simulink model "VCU_CS75_12_16_Test"  (R2014a)
settings: Solver=FixedStepDiscrete  StartTime=0.0  StopTime=25  FixedStep=0.0005  RelTol=1e-3
undefined symbols (not defined in the file): ecucoder_acal, I_SW01_L, LaterlAngleCommand, LDW, RemoteAcclPosition
libraries: simulink x913, ec5744lib x39
(part 25 of 30)

== system VCU_CS75_12_16_Test/长安CS75底盘程序，20ms一次/Input/CAN1_Rx/EMS_205/ReceiveMessages/Subsystem/EMS ==
  input : Inport
  Demux : Demux  Outputs=8
  EMS_CheckSum_205_Ad : Sum
  EMS_CheckSum_205_Convert : DataTypeConversion  OutDataTypeStr=uint32
  EMS_CheckSum_205_F : Gain
  EMS_CheckSum_205_L : simulink/Logic and Bit Operations/Bitwise Operator  logicop=AND  UseBitMask=on  BitMask=240  BitMaskRealWorld=Stored Integer
  EMS_CheckSum_205_O : Constant  Value=0  OutDataTypeStr=single
  EMS_CheckSum_205_S : ArithShift  BitShiftNumber=4
  EMS_CheckSum_205_Sub : Subsystem
  EMS_CheckSum_205_sat : Saturate  UpperLimit=15  LowerLimit=0
  EMS_CheckSum_205cv : DataTypeConversion
  EMS_ESPTorqReuestAvailability_Ad : Sum
  EMS_ESPTorqReuestAvailability_Convert : DataTypeConversion  OutDataTypeStr=uint32
  EMS_ESPTorqReuestAvailability_F : Gain
  EMS_ESPTorqReuestAvailability_L : simulink/Logic and Bit Operations/Bitwise Operator  logicop=AND  UseBitMask=on  BitMask=2  BitMaskRealWorld=Stored Integer
  EMS_ESPTorqReuestAvailability_O : Constant  Value=0  OutDataTypeStr=single
  EMS_ESPTorqReuestAvailability_S : ArithShift  BitShiftNumber=1
  EMS_ESPTorqReuestAvailability_Sub : Subsystem
  EMS_ESPTorqReuestAvailability_sat : Saturate  UpperLimit=1  LowerLimit=0  OutDataTypeStr=Inherit: Inherit via back propagation
  EMS_ESPTorqReuestAvailabilitycv : DataTypeConversion
  EMS_FrictionalTorq_Ad : Sum
  EMS_FrictionalTorq_Convert : DataTypeConversion  OutDataTypeStr=uint32
  EMS_FrictionalTorq_F : Gain  Gain=0.001526
  EMS_FrictionalTorq_L : simulink/Logic and Bit Operations/Bitwise Operator  logicop=AND  UseBitMask=on  BitMask=65535  BitMaskRealWorld=Stored Integer
  EMS_FrictionalTorq_O : Constant  Value=0  OutDataTypeStr=single
  EMS_FrictionalTorq_S : ArithShift
  EMS_FrictionalTorq_Sub : Subsystem
  EMS_FrictionalTorq_sat : Saturate  UpperLimit=99.9988  LowerLimit=0
  EMS_FrictionalTorqcv : DataTypeConversion
  EMS_FrictionalTorqinput4_Ad : Sum
  EMS_FrictionalTorqinput4_C : Constant  Value=256
  EMS_FrictionalTorqinput4_P : Product
  EMS_IndicatedDriverReqTorq_Ad : Sum
  EMS_IndicatedDriverReqTorq_Convert : DataTypeConversion  OutDataTypeStr=uint32
  EMS_IndicatedDriverReqTorq_F : Gain  Gain=0.001526
  EMS_IndicatedDriverReqTorq_L : simulink/Logic and Bit Operations/Bitwise Operator  logicop=AND  UseBitMask=on  BitMask=65535  BitMaskRealWorld=Stored Integer
  EMS_IndicatedDriverReqTorq_O : Constant  Value=0  OutDataTypeStr=single
  EMS_IndicatedDriverReqTorq_S : ArithShift
  EMS_IndicatedDriverReqTorq_Sub : Subsystem
  EMS_IndicatedDriverReqTorq_sat : Saturate  UpperLimit=99.9988  LowerLimit=0
  EMS_IndicatedDriverReqTorqcv : DataTypeConversion
  EMS_IndicatedDriverReqTorqinput2_Ad : Sum
  EMS_IndicatedDriverReqTorqinput2_C : Constant  Value=256
  EMS_IndicatedDriverReqTorqinput2_P : Product
  EMS_IndicatedRealEngTorq_Ad : Sum
  EMS_IndicatedRealEngTorq_Convert : DataTypeConversion  OutDataTypeStr=uint32
  EMS_IndicatedRealEngTorq_F : Gain  Gain=0.001526
  EMS_IndicatedRealEngTorq_L : simulink/Logic and Bit Operations/Bitwise Operator  logicop=AND  UseBitMask=on  BitMask=65535  BitMaskRealWorld=Stored Integer
  EMS_IndicatedRealEngTorq_O : Constant  Value=0  OutDataTypeStr=single
  EMS_IndicatedRealEngTorq_S : ArithShift
  EMS_IndicatedRealEngTorq_Sub : Subsystem
  EMS_IndicatedRealEngTorq_sat : Saturate  UpperLimit=99.9988  LowerLimit=0
  EMS_IndicatedRealEngTorqcv : DataTypeConversion
  EMS_IndicatedRealEngTorqinput6_Ad : Sum
  EMS_IndicatedRealEngTorqinput6_C : Constant  Value=256
  EMS_IndicatedRealEngTorqinput6_P : Product
  EMS_RollingCounter_id205_Ad : Sum
  EMS_RollingCounter_id205_Convert : DataTypeConversion  OutDataTypeStr=uint32
  EMS_RollingCounter_id205_F : Gain
  EMS_RollingCounter_id205_L : simulink/Logic and Bit Operations/Bitwise Operator  logicop=AND  UseBitMask=on  BitMask=15  BitMaskRealWorld=Stored Integer
  EMS_RollingCounter_id205_O : Constant  Value=0  OutDataTypeStr=single
  EMS_RollingCounter_id205_S : ArithShift
  EMS_RollingCounter_id205_Sub : Subsystem
  EMS_RollingCounter_id205_sat : Saturate  UpperLimit=15  LowerLimit=0
  EMS_RollingCounter_id205cv : DataTypeConversion
  EMS_TorqFailure_Ad : Sum
  EMS_TorqFailure_Convert : DataTypeConversion  OutDataTypeStr=uint32
  EMS_TorqFailure_F : Gain
  EMS_TorqFailure_L : simulink/Logic and Bit Operations/Bitwise Operator  logicop=AND  UseBitMask=on  BitMask=128  BitMaskRealWorld=Stored Integer
  EMS_TorqFailure_O : Constant  Value=0  OutDataTypeStr=single
  EMS_TorqFailure_S : ArithShift  BitShiftNumber=7
  EMS_TorqFailure_Sub : Subsystem
  EMS_TorqFailure_sat : Saturate  UpperLimit=1  LowerLimit=0
  EMS_TorqFailurecv : DataTypeConversion
  EMS_ESPTorqReuestAvailability_Out : Outport
  EMS_TorqFailure_Out : Outport  Port=2
  EMS_IndicatedDriverReqTorq_Out : Outport  Port=3
  EMS_FrictionalTorq_Out : Outport  Port=4
  EMS_IndicatedRealEngTorq_Out : Outport  Port=5
  EMS_RollingCounter_id205_Out : Outport  Port=6
  EMS_CheckSum_205_Out : Outport  Port=7
  wires:
  EMS_ESPTorqReuestAvailability_F/1 -> EMS_ESPTorqReuestAvailability_Ad/1
  EMS_ESPTorqReuestAvailability_O/1 -> EMS_ESPTorqReuestAvailability_Ad/2
  EMS_ESPTorqReuestAvailability_sat/1 -> EMS_ESPTorqReuestAvailability_Out/1
  Demux/1 -> EMS_ESPTorqReuestAvailability_Sub/1(In1), EMS_TorqFailure_Sub/1(In1)
  EMS_ESPTorqReuestAvailability_Sub/1(Out1) -> EMS_ESPTorqReuestAvailability_Convert/1
  EMS_ESPTorqReuestAvailability_Convert/1 -> EMS_ESPTorqReuestAvailability_L/1
  EMS_ESPTorqReuestAvailability_L/1 -> EMS_ESPTorqReuestAvailability_S/1
  EMS_ESPTorqReuestAvailability_S/1 -> EMS_ESPTorqReuestAvailabilitycv/1
  EMS_ESPTorqReuestAvailabilitycv/1 -> EMS_ESPTorqReuestAvailability_F/1
  EMS_TorqFailure_F/1 -> EMS_TorqFailure_Ad/1
  EMS_TorqFailure_O/1 -> EMS_TorqFailure_Ad/2
  EMS_TorqFailure_Ad/1 -> EMS_TorqFailure_sat/1
  EMS_TorqFailure_sat/1 -> EMS_TorqFailure_Out/1
  EMS_TorqFailure_Sub/1(Out1) -> EMS_TorqFailure_Convert/1
  EMS_TorqFailure_Convert/1 -> EMS_TorqFailure_L/1
  EMS_TorqFailure_L/1 -> EMS_TorqFailure_S/1
  EMS_TorqFailure_S/1 -> EMS_TorqFailurecv/1
  EMS_TorqFailurecv/1 -> EMS_TorqFailure_F/1
  EMS_IndicatedDriverReqTorq_F/1 -> EMS_IndicatedDriverReqTorq_Ad/1
  EMS_IndicatedDriverReqTorq_O/1 -> EMS_IndicatedDriverReqTorq_Ad/2
  EMS_IndicatedDriverReqTorq_Ad/1 -> EMS_IndicatedDriverReqTorq_sat/1
  EMS_IndicatedDriverReqTorq_sat/1 -> EMS_IndicatedDriverReqTorq_Out/1
  Demux/2 -> EMS_IndicatedDriverReqTorqinput2_P/1
  EMS_IndicatedDriverReqTorqinput2_C/1 -> EMS_IndicatedDriverReqTorqinput2_P/2
  EMS_IndicatedDriverReqTorqinput2_P/1 -> EMS_IndicatedDriverReqTorqinput2_Ad/1
  Demux/3 -> EMS_IndicatedDriverReqTorqinput2_Ad/2
  EMS_IndicatedDriverReqTorqinput2_Ad/1 -> EMS_IndicatedDriverReqTorq_Sub/1(In1)
  EMS_IndicatedDriverReqTorq_Sub/1(Out1) -> EMS_IndicatedDriverReqTorq_Convert/1
  EMS_IndicatedDriverReqTorq_Convert/1 -> EMS_IndicatedDriverReqTorq_L/1
  EMS_IndicatedDriverReqTorq_L/1 -> EMS_IndicatedDriverReqTorq_S/1
  EMS_IndicatedDriverReqTorq_S/1 -> EMS_IndicatedDriverReqTorqcv/1
  EMS_IndicatedDriverReqTorqcv/1 -> EMS_IndicatedDriverReqTorq_F/1
  EMS_FrictionalTorq_F/1 -> EMS_FrictionalTorq_Ad/1
  EMS_FrictionalTorq_O/1 -> EMS_FrictionalTorq_Ad/2
  EMS_FrictionalTorq_Ad/1 -> EMS_FrictionalTorq_sat/1
  EMS_FrictionalTorq_sat/1 -> EMS_FrictionalTorq_Out/1
  Demux/4 -> EMS_FrictionalTorqinput4_P/1
  EMS_FrictionalTorqinput4_C/1 -> EMS_FrictionalTorqinput4_P/2
  EMS_FrictionalTorqinput4_P/1 -> EMS_FrictionalTorqinput4_Ad/1
  Demux/5 -> EMS_FrictionalTorqinput4_Ad/2
  EMS_FrictionalTorqinput4_Ad/1 -> EMS_FrictionalTorq_Sub/1(In1)
  EMS_FrictionalTorq_Sub/1(Out1) -> EMS_FrictionalTorq_Convert/1
  EMS_FrictionalTorq_Convert/1 -> EMS_FrictionalTorq_L/1
  EMS_FrictionalTorq_L/1 -> EMS_FrictionalTorq_S/1
  EMS_FrictionalTorq_S/1 -> EMS_FrictionalTorqcv/1
  EMS_FrictionalTorqcv/1 -> EMS_FrictionalTorq_F/1
  EMS_IndicatedRealEngTorq_F/1 -> EMS_IndicatedRealEngTorq_Ad/1
  EMS_IndicatedRealEngTorq_O/1 -> EMS_IndicatedRealEngTorq_Ad/2
  EMS_IndicatedRealEngTorq_Ad/1 -> EMS_IndicatedRealEngTorq_sat/1
  EMS_IndicatedRealEngTorq_sat/1 -> EMS_IndicatedRealEngTorq_Out/1
  Demux/6 -> EMS_IndicatedRealEngTorqinput6_P/1
  EMS_IndicatedRealEngTorqinput6_C/1 -> EMS_IndicatedRealEngTorqinput6_P/2
  EMS_IndicatedRealEngTorqinput6_P/1 -> EMS_IndicatedRealEngTorqinput6_Ad/1
  Demux/7 -> EMS_IndicatedRealEngTorqinput6_Ad/2
  EMS_IndicatedRealEngTorqinput6_Ad/1 -> EMS_IndicatedRealEngTorq_Sub/1(In1)
  EMS_IndicatedRealEngTorq_Sub/1(Out1) -> EMS_IndicatedRealEngTorq_Convert/1
  EMS_IndicatedRealEngTorq_Convert/1 -> EMS_IndicatedRealEngTorq_L/1
  EMS_IndicatedRealEngTorq_L/1 -> EMS_IndicatedRealEngTorq_S/1
  EMS_IndicatedRealEngTorq_S/1 -> EMS_IndicatedRealEngTorqcv/1
  EMS_IndicatedRealEngTorqcv/1 -> EMS_IndicatedRealEngTorq_F/1
  EMS_RollingCounter_id205_F/1 -> EMS_RollingCounter_id205_Ad/1
  EMS_RollingCounter_id205_O/1 -> EMS_RollingCounter_id205_Ad/2
  EMS_RollingCounter_id205_Ad/1 -> EMS_RollingCounter_id205_sat/1
  EMS_RollingCounter_id205_sat/1 -> EMS_RollingCounter_id205_Out/1
  Demux/8 -> EMS_RollingCounter_id205_Sub/1(In1), EMS_CheckSum_205_Sub/1(In1)
  EMS_RollingCounter_id205_Sub/1(Out1) -> EMS_RollingCounter_id205_Convert/1
  EMS_RollingCounter_id205_Convert/1 -> EMS_RollingCounter_id205_L/1
  EMS_RollingCounter_id205_L/1 -> EMS_RollingCounter_id205_S/1
  EMS_RollingCounter_id205_S/1 -> EMS_RollingCounter_id205cv/1
  EMS_RollingCounter_id205cv/1 -> EMS_RollingCounter_id205_F/1
  EMS_CheckSum_205_F/1 -> EMS_CheckSum_205_Ad/1
  EMS_CheckSum_205_O/1 -> EMS_CheckSum_205_Ad/2
  EMS_CheckSum_205_Ad/1 -> EMS_CheckSum_205_sat/1
  EMS_CheckSum_205_sat/1 -> EMS_CheckSum_205_Out/1
  EMS_CheckSum_205_Sub/1(Out1) -> EMS_CheckSum_205_Convert/1
  EMS_CheckSum_205_Convert/1 -> EMS_CheckSum_205_L/1
  EMS_CheckSum_205_L/1 -> EMS_CheckSum_205_S/1
  EMS_CheckSum_205_S/1 -> EMS_CheckSum_205cv/1
  EMS_CheckSum_205cv/1 -> EMS_CheckSum_205_F/1
  input/1 -> Demux/1
  EMS_ESPTorqReuestAvailability_Ad/1 -> EMS_ESPTorqReuestAvailability_sat/1

== system VCU_CS75_12_16_Test/长安CS75底盘程序，20ms一次/Input/CAN1_Rx/EMS_255/ReceiveMessages/Subsystem/EMS ==
  input : Inport
  Demux : Demux  Outputs=8
  EMS_AccPedal_Ad : Sum
  EMS_AccPedal_Convert : DataTypeConversion  OutDataTypeStr=uint32
  EMS_AccPedal_F : Gain  Gain=0.392
  EMS_AccPedal_L : simulink/Logic and Bit Operations/Bitwise Operator  logicop=AND  UseBitMask=on  BitMask=255  BitMaskRealWorld=Stored Integer
  EMS_AccPedal_O : Constant  Value=0  OutDataTypeStr=single
  EMS_AccPedal_S : ArithShift
  EMS_AccPedal_Sub : Subsystem
  EMS_AccPedal_sat : Saturate  UpperLimit=99.568  LowerLimit=0
  EMS_AccPedalcv : DataTypeConversion
  EMS_AccpedelError_Ad : Sum
  EMS_AccpedelError_Convert : DataTypeConversion  OutDataTypeStr=uint32
  EMS_AccpedelError_F : Gain
  EMS_AccpedelError_L : simulink/Logic and Bit Operations/Bitwise Operator  logicop=AND  UseBitMask=on  BitMask=4  BitMaskRealWorld=Stored Integer
  EMS_AccpedelError_O : Constant  Value=0  OutDataTypeStr=single
  EMS_AccpedelError_S : ArithShift  BitShiftNumber=2
  EMS_AccpedelError_Sub : Subsystem
  EMS_AccpedelError_sat : Saturate  UpperLimit=1  LowerLimit=0
  EMS_AccpedelErrorcv : DataTypeConversion
  EMS_BrakePedalStatus_Ad : Sum
  EMS_BrakePedalStatus_Convert : DataTypeConversion  OutDataTypeStr=uint32
  EMS_BrakePedalStatus_F : Gain
  EMS_BrakePedalStatus_L : simulink/Logic and Bit Operations/Bitwise Operator  logicop=AND  UseBitMask=on  BitMask=192  BitMaskRealWorld=Stored Integer
  EMS_BrakePedalStatus_O : Constant  Value=0  OutDataTypeStr=single
  EMS_BrakePedalStatus_S : ArithShift  BitShiftNumber=6
  EMS_BrakePedalStatus_Sub : Subsystem
  EMS_BrakePedalStatus_sat : Saturate  UpperLimit=3  LowerLimit=0
  EMS_BrakePedalStatuscv : DataTypeConversion
  EMS_CheckSum_255_Ad : Sum
  EMS_CheckSum_255_Convert : DataTypeConversion  OutDataTypeStr=uint32
  EMS_CheckSum_255_F : Gain
  EMS_CheckSum_255_L : simulink/Logic and Bit Operations/Bitwise Operator  logicop=AND  UseBitMask=on  BitMask=240  BitMaskRealWorld=Stored Integer
  EMS_CheckSum_255_O : Constant  Value=0  OutDataTypeStr=single
  EMS_CheckSum_255_S : ArithShift  BitShiftNumber=4
  EMS_CheckSum_255_Sub : Subsystem
  EMS_CheckSum_255_sat : Saturate  UpperLimit=15  LowerLimit=0
  EMS_CheckSum_255cv : DataTypeConversion
  EMS_EngineSpeedError_Ad : Sum
  EMS_EngineSpeedError_Convert : DataTypeConversion  OutDataTypeStr=uint32
  EMS_EngineSpeedError_F : Gain
  EMS_EngineSpeedError_L : simulink/Logic and Bit Operations/Bitwise Operator  logicop=AND  UseBitMask=on  BitMask=16  BitMaskRealWorld=Stored Integer
  EMS_EngineSpeedError_O : Constant  Value=0  OutDataTypeStr=single
  EMS_EngineSpeedError_S : ArithShift  BitShiftNumber=4
  EMS_EngineSpeedError_Sub : Subsystem
  EMS_EngineSpeedError_sat : Saturate  UpperLimit=1  LowerLimit=0
  EMS_EngineSpeedErrorcv : DataTypeConversion
  EMS_EngineSpeed_Ad : Sum
  EMS_EngineSpeed_Convert : DataTypeConversion  OutDataTypeStr=uint32
  EMS_EngineSpeed_F : Gain  Gain=0.25
  EMS_EngineSpeed_L : simulink/Logic and Bit Operations/Bitwise Operator  logicop=AND  UseBitMask=on  BitMask=65535  BitMaskRealWorld=Stored Integer
  EMS_EngineSpeed_O : Constant  Value=0  OutDataTypeStr=single
  EMS_EngineSpeed_S : ArithShift
  EMS_EngineSpeed_Sub : Subsystem
  EMS_EngineSpeed_sat : Saturate  UpperLimit=16383.5  LowerLimit=0
  EMS_EngineSpeedcv : DataTypeConversion
  EMS_EngineSpeedinput3_Ad : Sum
  EMS_EngineSpeedinput3_C : Constant  Value=256
  EMS_EngineSpeedinput3_P : Product
  EMS_RollingCounter_id255_Ad : Sum
  EMS_RollingCounter_id255_Convert : DataTypeConversion  OutDataTypeStr=uint32
  EMS_RollingCounter_id255_F : Gain
  EMS_RollingCounter_id255_L : simulink/Logic and Bit Operations/Bitwise Operator  logicop=AND  UseBitMask=on  BitMask=15  BitMaskRealWorld=Stored Integer
  EMS_RollingCounter_id255_O : Constant  Value=0  OutDataTypeStr=single
  EMS_RollingCounter_id255_S : ArithShift
  EMS_RollingCounter_id255_Sub : Subsystem
  EMS_RollingCounter_id255_sat : Saturate  UpperLimit=15  LowerLimit=0
  EMS_RollingCounter_id255cv : DataTypeConversion
  EMS_BrakePedalStatus_Out : Outport
  EMS_AccpedelError_Out : Outport  Port=2
  EMS_EngineSpeedError_Out : Outport  Port=3
  EMS_EngineSpeed_Out : Outport  Port=4
  EMS_AccPedal_Out : Outport  Port=5
  EMS_RollingCounter_id255_Out : Outport  Port=6
  EMS_CheckSum_255_Out : Outport  Port=7
  wires:
  EMS_BrakePedalStatus_F/1 -> EMS_BrakePedalStatus_Ad/1
  EMS_BrakePedalStatus_O/1 -> EMS_BrakePedalStatus_Ad/2
  EMS_BrakePedalStatus_Ad/1 -> EMS_BrakePedalStatus_sat/1
  EMS_BrakePedalStatus_sat/1 -> EMS_BrakePedalStatus_Out/1
  Demux/1 -> EMS_BrakePedalStatus_Sub/1(In1)
  EMS_BrakePedalStatus_Sub/1(Out1) -> EMS_BrakePedalStatus_Convert/1
  EMS_BrakePedalStatus_Convert/1 -> EMS_BrakePedalStatus_L/1
  EMS_BrakePedalStatus_L/1 -> EMS_BrakePedalStatus_S/1
  EMS_BrakePedalStatus_S/1 -> EMS_BrakePedalStatuscv/1
  EMS_BrakePedalStatuscv/1 -> EMS_BrakePedalStatus_F/1
  EMS_AccpedelError_F/1 -> EMS_AccpedelError_Ad/1
  EMS_AccpedelError_O/1 -> EMS_AccpedelError_Ad/2
  EMS_AccpedelError_Ad/1 -> EMS_AccpedelError_sat/1
  EMS_AccpedelError_sat/1 -> EMS_AccpedelError_Out/1
  Demux/2 -> EMS_AccpedelError_Sub/1(In1), EMS_EngineSpeedError_Sub/1(In1)
  EMS_AccpedelError_Sub/1(Out1) -> EMS_AccpedelError_Convert/1
  EMS_AccpedelError_Convert/1 -> EMS_AccpedelError_L/1
  EMS_AccpedelError_L/1 -> EMS_AccpedelError_S/1
  EMS_AccpedelError_S/1 -> EMS_AccpedelErrorcv/1
  EMS_AccpedelErrorcv/1 -> EMS_AccpedelError_F/1
  EMS_EngineSpeedError_F/1 -> EMS_EngineSpeedError_Ad/1
  EMS_EngineSpeedError_O/1 -> EMS_EngineSpeedError_Ad/2
  EMS_EngineSpeedError_Ad/1 -> EMS_EngineSpeedError_sat/1
  EMS_EngineSpeedError_sat/1 -> EMS_EngineSpeedError_Out/1
  EMS_EngineSpeedError_Sub/1(Out1) -> EMS_EngineSpeedError_Convert/1
  EMS_EngineSpeedError_Convert/1 -> EMS_EngineSpeedError_L/1
  EMS_EngineSpeedError_L/1 -> EMS_EngineSpeedError_S/1
  EMS_EngineSpeedError_S/1 -> EMS_EngineSpeedErrorcv/1
  EMS_EngineSpeedErrorcv/1 -> EMS_EngineSpeedError_F/1
  EMS_EngineSpeed_F/1 -> EMS_EngineSpeed_Ad/1
  EMS_EngineSpeed_O/1 -> EMS_EngineSpeed_Ad/2
  EMS_EngineSpeed_Ad/1 -> EMS_EngineSpeed_sat/1
  EMS_EngineSpeed_sat/1 -> EMS_EngineSpeed_Out/1
  Demux/3 -> EMS_EngineSpeedinput3_P/1
  EMS_EngineSpeedinput3_C/1 -> EMS_EngineSpeedinput3_P/2
  EMS_EngineSpeedinput3_P/1 -> EMS_EngineSpeedinput3_Ad/1
  Demux/4 -> EMS_EngineSpeedinput3_Ad/2
  EMS_EngineSpeedinput3_Ad/1 -> EMS_EngineSpeed_Sub/1(In1)
  EMS_EngineSpeed_Sub/1(Out1) -> EMS_EngineSpeed_Convert/1
  EMS_EngineSpeed_Convert/1 -> EMS_EngineSpeed_L/1
  EMS_EngineSpeed_L/1 -> EMS_EngineSpeed_S/1
  EMS_EngineSpeed_S/1 -> EMS_EngineSpeedcv/1
  EMS_EngineSpeedcv/1 -> EMS_EngineSpeed_F/1
  EMS_AccPedal_F/1 -> EMS_AccPedal_Ad/1
  EMS_AccPedal_O/1 -> EMS_AccPedal_Ad/2
  EMS_AccPedal_Ad/1 -> EMS_AccPedal_sat/1
  EMS_AccPedal_sat/1 -> EMS_AccPedal_Out/1
  Demux/6 -> EMS_AccPedal_Sub/1(In1)
  EMS_AccPedal_Sub/1(Out1) -> EMS_AccPedal_Convert/1
  EMS_AccPedal_Convert/1 -> EMS_AccPedal_L/1
  EMS_AccPedal_L/1 -> EMS_AccPedal_S/1
  EMS_AccPedal_S/1 -> EMS_AccPedalcv/1
  EMS_AccPedalcv/1 -> EMS_AccPedal_F/1
  EMS_RollingCounter_id255_F/1 -> EMS_RollingCounter_id255_Ad/1
  EMS_RollingCounter_id255_O/1 -> EMS_RollingCounter_id255_Ad/2
  EMS_RollingCounter_id255_Ad/1 -> EMS_RollingCounter_id255_sat/1
  EMS_RollingCounter_id255_sat/1 -> EMS_RollingCounter_id255_Out/1
  Demux/8 -> EMS_RollingCounter_id255_Sub/1(In1), EMS_CheckSum_255_Sub/1(In1)
  EMS_RollingCounter_id255_Sub/1(Out1) -> EMS_RollingCounter_id255_Convert/1
  EMS_RollingCounter_id255_Convert/1 -> EMS_RollingCounter_id255_L/1
  EMS_RollingCounter_id255_L/1 -> EMS_RollingCounter_id255_S/1
  EMS_RollingCounter_id255_S/1 -> EMS_RollingCounter_id255cv/1
  EMS_RollingCounter_id255cv/1 -> EMS_RollingCounter_id255_F/1
  EMS_CheckSum_255_F/1 -> EMS_CheckSum_255_Ad/1
  EMS_CheckSum_255_O/1 -> EMS_CheckSum_255_Ad/2
  EMS_CheckSum_255_Ad/1 -> EMS_CheckSum_255_sat/1
  EMS_CheckSum_255_sat/1 -> EMS_CheckSum_255_Out/1
  EMS_CheckSum_255_Sub/1(Out1) -> EMS_CheckSum_255_Convert/1
  EMS_CheckSum_255_Convert/1 -> EMS_CheckSum_255_L/1
  EMS_CheckSum_255_L/1 -> EMS_CheckSum_255_S/1
  EMS_CheckSum_255_S/1 -> EMS_CheckSum_255cv/1
  EMS_CheckSum_255cv/1 -> EMS_CheckSum_255_F/1
  input/1 -> Demux/1

== system VCU_CS75_12_16_Test/长安CS75底盘程序，20ms一次/Input/CAN1_Rx/EMS_265/ReceiveMessages/Subsystem/EMS_265xx ==
  input : Inport
  Demux : Demux  Outputs=8
  EMS_EngineStatus_Ad : Sum
  EMS_EngineStatus_Convert : DataTypeConversion  OutDataTypeStr=uint32
  EMS_EngineStatus_F : Gain
  EMS_EngineStatus_L : simulink/Logic and Bit Operations/Bitwise Operator  logicop=AND  UseBitMask=on  BitMask=192  BitMaskRealWorld=Stored Integer
  EMS_EngineStatus_O : Constant  Value=0  OutDataTypeStr=single
  EMS_EngineStatus_S : ArithShift  BitShiftNumber=6
  EMS_EngineStatus_Sub : Subsystem
  EMS_EngineStatus_sat : Saturate  UpperLimit=3  LowerLimit=0
  EMS_EngineStatuscv : DataTypeConversion
  EMS_FullLoadIndicatedTorq_Ad : Sum
  EMS_FullLoadIndicatedTorq_Convert : DataTypeConversion  OutDataTypeStr=uint32
  EMS_FullLoadIndicatedTorq_F : Gain  Gain=0.392
  EMS_FullLoadIndicatedTorq_L : simulink/Logic and Bit Operations/Bitwise Operator  logicop=AND  UseBitMask=on  BitMask=255  BitMaskRealWorld=Stored Integer
  EMS_FullLoadIndicatedTorq_O : Constant  Value=0  OutDataTypeStr=single
  EMS_FullLoadIndicatedTorq_S : ArithShift
  EMS_FullLoadIndicatedTorq_Sub : Subsystem
  EMS_FullLoadIndicatedTorq_sat : Saturate  UpperLimit=99.96  LowerLimit=0
  EMS_FullLoadIndicatedTorqcv : DataTypeConversion
  EMS_RollingCounter_id265_Ad : Sum
  EMS_RollingCounter_id265_Convert : DataTypeConversion  OutDataTypeStr=uint32
  EMS_RollingCounter_id265_F : Gain
  EMS_RollingCounter_id265_L : simulink/Logic and Bit Operations/Bitwise Operator  logicop=AND  UseBitMask=on  BitMask=15  BitMaskRealWorld=Stored Integer
  EMS_RollingCounter_id265_O : Constant  Value=0  OutDataTypeStr=single
  EMS_RollingCounter_id265_S : ArithShift
  EMS_RollingCounter_id265_Sub : Subsystem
  EMS_RollingCounter_id265_sat : Saturate  UpperLimit=15  LowerLimit=0
  EMS_RollingCounter_id265cv : DataTypeConversion
  EMS_TorqueConstant_Ad : Sum
  EMS_TorqueConstant_Convert : DataTypeConversion  OutDataTypeStr=uint32
  EMS_TorqueConstant_F : Gain  Gain=10
  EMS_TorqueConstant_L : simulink/Logic and Bit Operations/Bitwise Operator  logicop=AND  UseBitMask=on  BitMask=255  BitMaskRealWorld=Stored Integer
  EMS_TorqueConstant_O : Constant  Value=0  OutDataTypeStr=single
  EMS_TorqueConstant_S : ArithShift
  EMS_TorqueConstant_Sub : Subsystem
  EMS_TorqueConstant_sat : Saturate  UpperLimit=2540  LowerLimit=0
  EMS_TorqueConstantcv : DataTypeConversion
  EMS_FullLoadIndicatedTorq_Out : Outport
  EMS_TorqueConstant_Out : Outport  Port=2
  EMS_RollingCounter_id265_Out : Outport  Port=3
  EMS_EngineStatus_Out : Outport  Port=4
  wires:
  EMS_FullLoadIndicatedTorq_F/1 -> EMS_FullLoadIndicatedTorq_Ad/1
  EMS_FullLoadIndicatedTorq_O/1 -> EMS_FullLoadIndicatedTorq_Ad/2
  EMS_FullLoadIndicatedTorq_Ad/1 -> EMS_FullLoadIndicatedTorq_sat/1
  EMS_FullLoadIndicatedTorq_sat/1 -> EMS_FullLoadIndicatedTorq_Out/1
  Demux/3 -> EMS_FullLoadIndicatedTorq_Sub/1(In1)
  EMS_FullLoadIndicatedTorq_Sub/1(Out1) -> EMS_FullLoadIndicatedTorq_Convert/1
  EMS_FullLoadIndicatedTorq_Convert/1 -> EMS_FullLoadIndicatedTorq_L/1
  EMS_FullLoadIndicatedTorq_L/1 -> EMS_FullLoadIndicatedTorq_S/1
  EMS_FullLoadIndicatedTorq_S/1 -> EMS_FullLoadIndicatedTorqcv/1
  EMS_FullLoadIndicatedTorqcv/1 -> EMS_FullLoadIndicatedTorq_F/1
  EMS_TorqueConstant_F/1 -> EMS_TorqueConstant_Ad/1
  EMS_TorqueConstant_O/1 -> EMS_TorqueConstant_Ad/2
  EMS_TorqueConstant_Ad/1 -> EMS_TorqueConstant_sat/1
  EMS_TorqueConstant_sat/1 -> EMS_TorqueConstant_Out/1
  Demux/7 -> EMS_TorqueConstant_Sub/1(In1)
  EMS_TorqueConstant_Sub/1(Out1) -> EMS_TorqueConstant_Convert/1
  EMS_TorqueConstant_Convert/1 -> EMS_TorqueConstant_L/1
  EMS_TorqueConstant_L/1 -> EMS_TorqueConstant_S/1
  EMS_TorqueConstant_S/1 -> EMS_TorqueConstantcv/1
  EMS_TorqueConstantcv/1 -> EMS_TorqueConstant_F/1
  EMS_RollingCounter_id265_F/1 -> EMS_RollingCounter_id265_Ad/1
  EMS_RollingCounter_id265_O/1 -> EMS_RollingCounter_id265_Ad/2
  EMS_RollingCounter_id265_Ad/1 -> EMS_RollingCounter_id265_sat/1
  EMS_RollingCounter_id265_sat/1 -> EMS_RollingCounter_id265_Out/1
  Demux/8 -> EMS_RollingCounter_id265_Sub/1(In1), EMS_EngineStatus_Sub/1(In1)
  EMS_RollingCounter_id265_Sub/1(Out1) -> EMS_RollingCounter_id265_Convert/1
  EMS_RollingCounter_id265_Convert/1 -> EMS_RollingCounter_id265_L/1
  EMS_RollingCounter_id265_L/1 -> EMS_RollingCounter_id265_S/1
  EMS_RollingCounter_id265_S/1 -> EMS_RollingCounter_id265cv/1
  EMS_RollingCounter_id265cv/1 -> EMS_RollingCounter_id265_F/1
  EMS_EngineStatus_F/1 -> EMS_EngineStatus_Ad/1
  EMS_EngineStatus_O/1 -> EMS_EngineStatus_Ad/2
  EMS_EngineStatus_Ad/1 -> EMS_EngineStatus_sat/1
  EMS_EngineStatus_sat/1 -> EMS_EngineStatus_Out/1
  EMS_EngineStatus_Sub/1(Out1) -> EMS_EngineStatus_Convert/1
  EMS_EngineStatus_Convert/1 -> EMS_EngineStatus_L/1
  EMS_EngineStatus_L/1 -> EMS_EngineStatus_S/1
  EMS_EngineStatus_S/1 -> EMS_EngineStatuscv/1
  EMS_EngineStatuscv/1 -> EMS_EngineStatus_F/1
  input/1 -> Demux/1

== system VCU_CS75_12_16_Test/长安CS75底盘程序，20ms一次/Input/CAN1_Rx/EMS_276/ReceiveMessages/Subsystem/EMS_2 ==
  input : Inport
  Demux : Demux  Outputs=8
  EMS_RealAccPedal_Ad : Sum
  EMS_RealAccPedal_Convert : DataTypeConversion  OutDataTypeStr=uint32
  EMS_RealAccPedal_F : Gain  Gain=0.392
  EMS_RealAccPedal_L : simulink/Logic and Bit Operations/Bitwise Operator  logicop=AND  UseBitMask=on  BitMask=255  BitMaskRealWorld=Stored Integer
  EMS_RealAccPedal_O : Constant  Value=0  OutDataTypeStr=single
  EMS_RealAccPedal_S : ArithShift
  EMS_RealAccPedal_Sub : Subsystem
  EMS_RealAccPedal_sat : Saturate  UpperLimit=99.96  LowerLimit=0
  EMS_RealAccPedalcv : DataTypeConversion
  EMS_RealAccPedal_Out : Outport
  wires:
  input/1 -> Demux/1
  EMS_RealAccPedalcv/1 -> EMS_RealAccPedal_F/1
  EMS_RealAccPedal_S/1 -> EMS_RealAccPedalcv/1
  EMS_RealAccPedal_L/1 -> EMS_RealAccPedal_S/1
  EMS_RealAccPedal_Convert/1 -> EMS_RealAccPedal_L/1
  EMS_RealAccPedal_Sub/1(Out1) -> EMS_RealAccPedal_Convert/1
  Demux/3 -> EMS_RealAccPedal_Sub/1(In1)
  EMS_RealAccPedal_sat/1 -> EMS_RealAccPedal_Out/1
  EMS_RealAccPedal_Ad/1 -> EMS_RealAccPedal_sat/1
  EMS_RealAccPedal_O/1 -> EMS_RealAccPedal_Ad/2
  EMS_RealAccPedal_F/1 -> EMS_RealAccPedal_Ad/1

== system VCU_CS75_12_16_Test/长安CS75底盘程序，20ms一次/Input/CAN1_Rx/EPB_256/ReceiveMessages/Subsystem/EPB ==
  input : Inport
  Demux : Demux  Outputs=8
  EPB_Checksum_Ad : Sum
  EPB_Checksum_Convert : DataTypeConversion  OutDataTypeStr=uint32
  EPB_Checksum_F : Gain
  EPB_Checksum_L : simulink/Logic and Bit Operations/Bitwise Operator  logicop=AND  UseBitMask=on  BitMask=255  BitMaskRealWorld=Stored Integer
  EPB_Checksum_O : Constant  Value=0  OutDataTypeStr=single
  EPB_Checksum_S : ArithShift
  EPB_Checksum_Sub : Subsystem
  EPB_Checksum_sat : Saturate  UpperLimit=255  LowerLimit=0
  EPB_Checksumcv : DataTypeConversion
  EPB_FailStatus_Ad : Sum
  EPB_FailStatus_Convert : DataTypeConversion  OutDataTypeStr=uint32
  EPB_FailStatus_F : Gain
  EPB_FailStatus_L : simulink/Logic and Bit Operations/Bitwise Operator  logicop=AND  UseBitMask=on  BitMask=192  BitMaskRealWorld=Stored Integer
  EPB_FailStatus_O : Constant  Value=0  OutDataTypeStr=single
  EPB_FailStatus_S : ArithShift  BitShiftNumber=6
  EPB_FailStatus_Sub : Subsystem
  EPB_FailStatus_sat : Saturate  UpperLimit=3  LowerLimit=0
  EPB_FailStatuscv : DataTypeConversion
  EPB_FailureLamp_Ad : Sum
  EPB_FailureLamp_Convert : DataTypeConversion  OutDataTypeStr=uint32
  EPB_FailureLamp_F : Gain
  EPB_FailureLamp_L : simulink/Logic and Bit Operations/Bitwise Operator  logicop=AND  UseBitMask=on  BitMask=48  BitMaskRealWorld=Stored Integer
  EPB_FailureLamp_O : Constant  Value=0  OutDataTypeStr=single
  EPB_FailureLamp_S : ArithShift  BitShiftNumber=4
  EPB_FailureLamp_Sub : Subsystem
  EPB_FailureLamp_sat : Saturate  UpperLimit=3  LowerLimit=0
  EPB_FailureLampcv : DataTypeConversion
  EPB_FunctionLamp_Ad : Sum
  EPB_FunctionLamp_Convert : DataTypeConversion  OutDataTypeStr=uint32
  EPB_FunctionLamp_F : Gain
  EPB_FunctionLamp_L : simulink/Logic and Bit Operations/Bitwise Operator  logicop=AND  UseBitMask=on  BitMask=12  BitMaskRealWorld=Stored Integer
  EPB_FunctionLamp_O : Constant  Value=0  OutDataTypeStr=single
  EPB_FunctionLamp_S : ArithShift  BitShiftNumber=2
  EPB_FunctionLamp_Sub : Subsystem
  EPB_FunctionLamp_sat : Saturate  UpperLimit=3  LowerLimit=0
  EPB_FunctionLampcv : DataTypeConversion
  EPB_RollingCounter_id256_Ad : Sum
  EPB_RollingCounter_id256_Convert : DataTypeConversion  OutDataTypeStr=uint32
  EPB_RollingCounter_id256_F : Gain
  EPB_RollingCounter_id256_L : simulink/Logic and Bit Operations/Bitwise Operator  logicop=AND  UseBitMask=on  BitMask=15  BitMaskRealWorld=Stored Integer
  EPB_RollingCounter_id256_O : Constant  Value=0  OutDataTypeStr=single
  EPB_RollingCounter_id256_S : ArithShift
  EPB_RollingCounter_id256_Sub : Subsystem
  EPB_RollingCounter_id256_sat : Saturate  UpperLimit=15  LowerLimit=0
  EPB_RollingCounter_id256cv : DataTypeConversion
  EPB_Status_Ad : Sum
  EPB_Status_Convert : DataTypeConversion  OutDataTypeStr=uint32
  EPB_Status_F : Gain
  EPB_Status_L : simulink/Logic and Bit Operations/Bitwise Operator  logicop=AND  UseBitMask=on  BitMask=192  BitMaskRealWorld=Stored Integer
  EPB_Status_O : Constant  Value=0  OutDataTypeStr=single
  EPB_Status_S : ArithShift  BitShiftNumber=6
  EPB_Status_Sub : Subsystem
  EPB_Status_sat : Saturate  UpperLimit=3  LowerLimit=0
  EPB_Statuscv : DataTypeConversion
  EPB_FailStatus_Out : Outport
  EPB_Status_Out : Outport  Port=2
  EPB_FunctionLamp_Out : Outport  Port=3
  EPB_FailureLamp_Out : Outport  Port=4
  EPB_RollingCounter_id256_Out : Outport  Port=5
  EPB_Checksum_Out : Outport  Port=6
  wires:
  EPB_FailStatus_F/1 -> EPB_FailStatus_Ad/1
  EPB_FailStatus_O/1 -> EPB_FailStatus_Ad/2
  EPB_FailStatus_Ad/1 -> EPB_FailStatus_sat/1
  EPB_FailStatus_sat/1 -> EPB_FailStatus_Out/1
  Demux/1 -> EPB_FailStatus_Sub/1(In1)
  EPB_FailStatus_Sub/1(Out1) -> EPB_FailStatus_Convert/1
  EPB_FailStatus_Convert/1 -> EPB_FailStatus_L/1
  EPB_FailStatus_L/1 -> EPB_FailStatus_S/1
  EPB_FailStatus_S/1 -> EPB_FailStatuscv/1
  EPB_FailStatuscv/1 -> EPB_FailStatus_F/1
  EPB_Status_F/1 -> EPB_Status_Ad/1
  EPB_Status_O/1 -> EPB_Status_Ad/2
  EPB_Status_Ad/1 -> EPB_Status_sat/1
  EPB_Status_sat/1 -> EPB_Status_Out/1
  Demux/3 -> EPB_Status_Sub/1(In1)
  EPB_Status_Sub/1(Out1) -> EPB_Status_Convert/1
  EPB_Status_Convert/1 -> EPB_Status_L/1
  EPB_Status_L/1 -> EPB_Status_S/1
  EPB_Status_S/1 -> EPB_Statuscv/1
  EPB_Statuscv/1 -> EPB_Status_F/1
  EPB_FunctionLamp_F/1 -> EPB_FunctionLamp_Ad/1
  EPB_FunctionLamp_O/1 -> EPB_FunctionLamp_Ad/2
  EPB_FunctionLamp_Ad/1 -> EPB_FunctionLamp_sat/1
  EPB_FunctionLamp_sat/1 -> EPB_FunctionLamp_Out/1
  Demux/6 -> EPB_FunctionLamp_Sub/1(In1), EPB_FailureLamp_Sub/1(In1)
  EPB_FunctionLamp_Sub/1(Out1) -> EPB_FunctionLamp_Convert/1
  EPB_FunctionLamp_Convert/1 -> EPB_FunctionLamp_L/1
  EPB_FunctionLamp_L/1 -> EPB_FunctionLamp_S/1
  EPB_FunctionLamp_S/1 -> EPB_FunctionLampcv/1
  EPB_FunctionLampcv/1 -> EPB_FunctionLamp_F/1
  EPB_FailureLamp_F/1 -> EPB_FailureLamp_Ad/1
  EPB_FailureLamp_O/1 -> EPB_FailureLamp_Ad/2
  EPB_FailureLamp_Ad/1 -> EPB_FailureLamp_sat/1
  EPB_FailureLamp_sat/1 -> EPB_FailureLamp_Out/1
  EPB_FailureLamp_Sub/1(Out1) -> EPB_FailureLamp_Convert/1
  EPB_FailureLamp_Convert/1 -> EPB_FailureLamp_L/1
  EPB_FailureLamp_L/1 -> EPB_FailureLamp_S/1
  EPB_FailureLamp_S/1 -> EPB_FailureLampcv/1
  EPB_FailureLampcv/1 -> EPB_FailureLamp_F/1
  EPB_RollingCounter_id256_F/1 -> EPB_RollingCounter_id256_Ad/1
  EPB_RollingCounter_id256_O/1 -> EPB_RollingCounter_id256_Ad/2
  EPB_RollingCounter_id256_Ad/1 -> EPB_RollingCounter_id256_sat/1
  EPB_RollingCounter_id256_sat/1 -> EPB_RollingCounter_id256_Out/1
  Demux/7 -> EPB_RollingCounter_id256_Sub/1(In1)
  EPB_RollingCounter_id256_Sub/1(Out1) -> EPB_RollingCounter_id256_Convert/1
  EPB_RollingCounter_id256_Convert/1 -> EPB_RollingCounter_id256_L/1
  EPB_RollingCounter_id256_L/1 -> EPB_RollingCounter_id256_S/1
  EPB_RollingCounter_id256_S/1 -> EPB_RollingCounter_id256cv/1
  EPB_RollingCounter_id256cv/1 -> EPB_RollingCounter_id256_F/1
  EPB_Checksum_F/1 -> EPB_Checksum_Ad/1
  EPB_Checksum_O/1 -> EPB_Checksum_Ad/2
  EPB_Checksum_Ad/1 -> EPB_Checksum_sat/1
  EPB_Checksum_sat/1 -> EPB_Checksum_Out/1
  Demux/8 -> EPB_Checksum_Sub/1(In1)
  EPB_Checksum_Sub/1(Out1) -> EPB_Checksum_Convert/1
  EPB_Checksum_Convert/1 -> EPB_Checksum_L/1
  EPB_Checksum_L/1 -> EPB_Checksum_S/1
  EPB_Checksum_S/1 -> EPB_Checksumcv/1
  EPB_Checksumcv/1 -> EPB_Checksum_F/1
  input/1 -> Demux/1

== system VCU_CS75_12_16_Test/长安CS75底盘程序，20ms一次/Input/CAN1_Rx/EPS_20A/ReceiveMessages/Subsystem/EPS_20A1 ==
  input : Inport
  Demux : Demux  Outputs=8
  EPS_APA_AbortFeedback_Ad : Sum
  EPS_APA_AbortFeedback_Convert : DataTypeConversion  OutDataTypeStr=uint32
  EPS_APA_AbortFeedback_F : Gain
  EPS_APA_AbortFeedback_L : simulink/Logic and Bit Operations/Bitwise Operator  logicop=AND  UseBitMask=on  BitMask=112  BitMaskRealWorld=Stored Integer
  EPS_APA_AbortFeedback_O : Constant  Value=0  OutDataTypeStr=single
  EPS_APA_AbortFeedback_S : ArithShift  BitShiftNumber=4
  EPS_APA_AbortFeedback_Sub : Subsystem
  EPS_APA_AbortFeedback_sat : Saturate  UpperLimit=7  LowerLimit=0
  EPS_APA_AbortFeedbackcv : DataTypeConversion
  EPS_APA_ControlFeedback_Ad : Sum
  EPS_APA_ControlFeedback_Convert : DataTypeConversion  OutDataTypeStr=uint32
  EPS_APA_ControlFeedback_F : Gain
  EPS_APA_ControlFeedback_L : simulink/Logic and Bit Operations/Bitwise Operator  logicop=AND  UseBitMask=on  BitMask=64  BitMaskRealWorld=Stored Integer
  EPS_APA_ControlFeedback_O : Constant  Value=0  OutDataTypeStr=single
  EPS_APA_ControlFeedback_S : ArithShift  BitShiftNumber=6
  EPS_APA_ControlFeedback_Sub : Subsystem
  EPS_APA_ControlFeedback_sat : Saturate  UpperLimit=1  LowerLimit=0
  EPS_APA_ControlFeedbackcv : DataTypeConversion
  EPS_APA_EpasFailed_Ad : Sum
  EPS_APA_EpasFailed_Convert : DataTypeConversion  OutDataTypeStr=uint32
  EPS_APA_EpasFailed_F : Gain
  EPS_APA_EpasFailed_L : simulink/Logic and Bit Operations/Bitwise Operator  logicop=AND  UseBitMask=on  BitMask=2  BitMaskRealWorld=Stored Integer
  EPS_APA_EpasFailed_O : Constant  Value=0  OutDataTypeStr=single
  EPS_APA_EpasFailed_S : ArithShift  BitShiftNumber=1
  EPS_APA_EpasFailed_Sub : Subsystem
  EPS_APA_EpasFailed_sat : Saturate  UpperLimit=1  LowerLimit=0
  EPS_APA_EpasFailedcv : DataTypeConversion
  EPS_Checksum_Ad : Sum
  EPS_Checksum_Convert : DataTypeConversion  OutDataTypeStr=uint32
  EPS_Checksum_F : Gain
  EPS_Checksum_L : simulink/Logic and Bit Operations/Bitwise Operator  logicop=AND  UseBitMask=on  BitMask=255  BitMaskRealWorld=Stored Integer
  EPS_Checksum_O : Constant  Value=0  OutDataTypeStr=single
  EPS_Checksum_S : ArithShift
  EPS_Checksum_Sub : Subsystem
  EPS_Checksum_sat : Saturate  UpperLimit=255  LowerLimit=0
  EPS_Checksumcv : DataTypeConversion
  EPS_ConcussAvailabilityStatus_Ad : Sum
  EPS_ConcussAvailabilityStatus_Convert : DataTypeConversion  OutDataTypeStr=uint32
  EPS_ConcussAvailabilityStatus_F : Gain
  EPS_ConcussAvailabilityStatus_L : simulink/Logic and Bit Operations/Bitwise Operator  logicop=AND  UseBitMask=on  BitMask=48  BitMaskRealWorld=Stored Integer
  EPS_ConcussAvailabilityStatus_O : Constant  Value=0  OutDataTypeStr=single
  EPS_ConcussAvailabilityStatus_S : ArithShift  BitShiftNumber=4
  EPS_ConcussAvailabilityStatus_Sub : Subsystem
  EPS_ConcussAvailabilityStatus_sat : Saturate  UpperLimit=3  LowerLimit=0
  EPS_ConcussAvailabilityStatuscv : DataTypeConversion
  EPS_EPSFailed_Ad : Sum
  EPS_EPSFailed_Convert : DataTypeConversion  OutDataTypeStr=uint32
  EPS_EPSFailed_F : Gain
  EPS_EPSFailed_L : simulink/Logic and Bit Operations/Bitwise Operator  logicop=AND  UseBitMask=on  BitMask=128  BitMaskRealWorld=Stored Integer
  EPS_EPSFailed_O : Constant  Value=0  OutDataTypeStr=single
  EPS_EPSFailed_S : ArithShift  BitShiftNumber=7
  EPS_EPSFailed_Sub : Subsystem
  EPS_EPSFailed_sat : Saturate  UpperLimit=1  LowerLimit=0
  EPS_EPSFailedcv : DataTypeConversion
  EPS_RollingCounter_Ad : Sum
  EPS_RollingCounter_Convert : DataTypeConversion  OutDataTypeStr=uint32
  EPS_RollingCounter_F : Gain
  EPS_RollingCounter_L : simulink/Logic and Bit Operations/Bitwise Operator  logicop=AND  UseBitMask=on  BitMask=15  BitMaskRealWorld=Stored Integer
  EPS_RollingCounter_O : Constant  Value=0  OutDataTypeStr=single
  EPS_RollingCounter_S : ArithShift
  EPS_RollingCounter_Sub : Subsystem
  EPS_RollingCounter_sat : Saturate  UpperLimit=15  LowerLimit=0
  EPS_RollingCountercv : DataTypeConversion
  EPS_SteeringTorque_Ad : Sum
  EPS_SteeringTorque_Convert : DataTypeConversion  OutDataTypeStr=uint32
  EPS_SteeringTorque_F : Gain  Gain=0.1794
  EPS_SteeringTorque_L : simulink/Logic and Bit Operations/Bitwise Operator  logicop=AND  UseBitMask=on  BitMask=4080  BitMaskRealWorld=Stored Integer
  EPS_SteeringTorque_O : Constant  Value=-22.78  OutDataTypeStr=single
  EPS_SteeringTorque_S : ArithShift  BitShiftNumber=4
  EPS_SteeringTorque_Sub : Subsystem
  EPS_SteeringTorque_sat : Saturate  UpperLimit=22.78  LowerLimit=-22.78
  EPS_SteeringTorquecv : DataTypeConversion
  EPS_SteeringTorqueinput3_Ad : Sum
  EPS_SteeringTorqueinput3_C : Constant  Value=256
  EPS_SteeringTorqueinput3_P : Product
  EPS_TorqueSensorStatus_Ad : Sum
  EPS_TorqueSensorStatus_Convert : DataTypeConversion  OutDataTypeStr=uint32
  EPS_TorqueSensorStatus_F : Gain
  EPS_TorqueSensorStatus_L : simulink/Logic and Bit Operations/Bitwise Operator  logicop=AND  UseBitMask=on  BitMask=2  BitMaskRealWorld=Stored Integer
  EPS_TorqueSensorStatus_O : Constant  Value=0  OutDataTypeStr=single
  EPS_TorqueSensorStatus_S : ArithShift  BitShiftNumber=1
  EPS_TorqueSensorStatus_Sub : Subsystem
  EPS_TorqueSensorStatus_sat : Saturate  UpperLimit=1  LowerLimit=0
  EPS_TorqueSensorStatuscv : DataTypeConversion
  EPS_EPSFailed_Out : Outport
  EPS_APA_EpasFailed_Out : Outport  Port=2
  EPS_APA_AbortFeedback_Out : Outport  Port=3
  EPS_SteeringTorque_Out : Outport  Port=4
  EPS_TorqueSensorStatus_Out : Outport  Port=5
  EPS_APA_ControlFeedback_Out : Outport  Port=6
  EPS_RollingCounter_Out : Outport  Port=7
  EPS_ConcussAvailabilityStatus_Out : Outport  Port=8
  EPS_Checksum_Out : Outport  Port=9
  wires:
  EPS_EPSFailed_F/1 -> EPS_EPSFailed_Ad/1
  EPS_EPSFailed_O/1 -> EPS_EPSFailed_Ad/2
  EPS_EPSFailed_Ad/1 -> EPS_EPSFailed_sat/1
  EPS_EPSFailed_sat/1 -> EPS_EPSFailed_Out/1
  Demux/1 -> EPS_EPSFailed_Sub/1(In1)
  EPS_EPSFailed_Sub/1(Out1) -> EPS_EPSFailed_Convert/1
  EPS_EPSFailed_Convert/1 -> EPS_EPSFailed_L/1
  EPS_EPSFailed_L/1 -> EPS_EPSFailed_S/1
  EPS_EPSFailed_S/1 -> EPS_EPSFailedcv/1
  EPS_EPSFailedcv/1 -> EPS_EPSFailed_F/1
  EPS_APA_EpasFailed_F/1 -> EPS_APA_EpasFailed_Ad/1
  EPS_APA_EpasFailed_O/1 -> EPS_APA_EpasFailed_Ad/2
  EPS_APA_EpasFailed_Ad/1 -> EPS_APA_EpasFailed_sat/1
  EPS_APA_EpasFailed_sat/1 -> EPS_APA_EpasFailed_Out/1
  Demux/2 -> EPS_APA_EpasFailed_Sub/1(In1), EPS_APA_AbortFeedback_Sub/1(In1)
  EPS_APA_EpasFailed_Sub/1(Out1) -> EPS_APA_EpasFailed_Convert/1
  EPS_APA_EpasFailed_Convert/1 -> EPS_APA_EpasFailed_L/1
  EPS_APA_EpasFailed_L/1 -> EPS_APA_EpasFailed_S/1
  EPS_APA_EpasFailed_S/1 -> EPS_APA_EpasFailedcv/1
  EPS_APA_EpasFailedcv/1 -> EPS_APA_EpasFailed_F/1
  EPS_APA_AbortFeedback_F/1 -> EPS_APA_AbortFeedback_Ad/1
  EPS_APA_AbortFeedback_O/1 -> EPS_APA_AbortFeedback_Ad/2
  EPS_APA_AbortFeedback_Ad/1 -> EPS_APA_AbortFeedback_sat/1
  EPS_APA_AbortFeedback_sat/1 -> EPS_APA_AbortFeedback_Out/1
  EPS_APA_AbortFeedback_Sub/1(Out1) -> EPS_APA_AbortFeedback_Convert/1
  EPS_APA_AbortFeedback_Convert/1 -> EPS_APA_AbortFeedback_L/1
  EPS_APA_AbortFeedback_L/1 -> EPS_APA_AbortFeedback_S/1
  EPS_APA_AbortFeedback_S/1 -> EPS_APA_AbortFeedbackcv/1
  EPS_APA_AbortFeedbackcv/1 -> EPS_APA_AbortFeedback_F/1
  EPS_SteeringTorque_F/1 -> EPS_SteeringTorque_Ad/1
  EPS_SteeringTorque_O/1 -> EPS_SteeringTorque_Ad/2
  EPS_SteeringTorque_Ad/1 -> EPS_SteeringTorque_sat/1
  EPS_SteeringTorque_sat/1 -> EPS_SteeringTorque_Out/1
  Demux/3 -> EPS_SteeringTorqueinput3_P/1
  EPS_SteeringTorqueinput3_C/1 -> EPS_SteeringTorqueinput3_P/2
  EPS_SteeringTorqueinput3_P/1 -> EPS_SteeringTorqueinput3_Ad/1
  Demux/4 -> EPS_SteeringTorqueinput3_Ad/2
  EPS_SteeringTorqueinput3_Ad/1 -> EPS_SteeringTorque_Sub/1(In1)
  EPS_SteeringTorque_Sub/1(Out1) -> EPS_SteeringTorque_Convert/1
  EPS_SteeringTorque_Convert/1 -> EPS_SteeringTorque_L/1
  EPS_SteeringTorque_L/1 -> EPS_SteeringTorque_S/1
  EPS_SteeringTorque_S/1 -> EPS_SteeringTorquecv/1
  EPS_SteeringTorquecv/1 -> EPS_SteeringTorque_F/1
  EPS_TorqueSensorStatus_F/1 -> EPS_TorqueSensorStatus_Ad/1
  EPS_TorqueSensorStatus_O/1 -> EPS_TorqueSensorStatus_Ad/2
  EPS_TorqueSensorStatus_Ad/1 -> EPS_TorqueSensorStatus_sat/1
  EPS_TorqueSensorStatus_sat/1 -> EPS_TorqueSensorStatus_Out/1
  Demux/5 -> EPS_TorqueSensorStatus_Sub/1(In1)
  EPS_TorqueSensorStatus_Sub/1(Out1) -> EPS_TorqueSensorStatus_Convert/1
  EPS_TorqueSensorStatus_Convert/1 -> EPS_TorqueSensorStatus_L/1
  EPS_TorqueSensorStatus_L/1 -> EPS_TorqueSensorStatus_S/1
  EPS_TorqueSensorStatus_S/1 -> EPS_TorqueSensorStatuscv/1
  EPS_TorqueSensorStatuscv/1 -> EPS_TorqueSensorStatus_F/1
  EPS_APA_ControlFeedback_F/1 -> EPS_APA_ControlFeedback_Ad/1
  EPS_APA_ControlFeedback_O/1 -> EPS_APA_ControlFeedback_Ad/2
  EPS_APA_ControlFeedback_Ad/1 -> EPS_APA_ControlFeedback_sat/1
  EPS_APA_ControlFeedback_sat/1 -> EPS_APA_ControlFeedback_Out/1
  Demux/6 -> EPS_APA_ControlFeedback_Sub/1(In1)
  EPS_APA_ControlFeedback_Sub/1(Out1) -> EPS_APA_ControlFeedback_Convert/1
  EPS_APA_ControlFeedback_Convert/1 -> EPS_APA_ControlFeedback_L/1
  EPS_APA_ControlFeedback_L/1 -> EPS_APA_ControlFeedback_S/1
  EPS_APA_ControlFeedback_S/1 -> EPS_APA_ControlFeedbackcv/1
  EPS_APA_ControlFeedbackcv/1 -> EPS_APA_ControlFeedback_F/1
  EPS_RollingCounter_F/1 -> EPS_RollingCounter_Ad/1
  EPS_RollingCounter_O/1 -> EPS_RollingCounter_Ad/2
  EPS_RollingCounter_Ad/1 -> EPS_RollingCounter_sat/1
  EPS_RollingCounter_sat/1 -> EPS_RollingCounter_Out/1
  Demux/7 -> EPS_RollingCounter_Sub/1(In1), EPS_ConcussAvailabilityStatus_Sub/1(In1)
  EPS_RollingCounter_Sub/1(Out1) -> EPS_RollingCounter_Convert/1
  EPS_RollingCounter_Convert/1 -> EPS_RollingCounter_L/1
  EPS_RollingCounter_L/1 -> EPS_RollingCounter_S/1
  EPS_RollingCounter_S/1 -> EPS_RollingCountercv/1
  EPS_RollingCountercv/1 -> EPS_RollingCounter_F/1
  EPS_ConcussAvailabilityStatus_F/1 -> EPS_ConcussAvailabilityStatus_Ad/1
  EPS_ConcussAvailabilityStatus_O/1 -> EPS_ConcussAvailabilityStatus_Ad/2
  EPS_ConcussAvailabilityStatus_Ad/1 -> EPS_ConcussAvailabilityStatus_sat/1
  EPS_ConcussAvailabilityStatus_sat/1 -> EPS_ConcussAvailabilityStatus_Out/1
  EPS_ConcussAvailabilityStatus_Sub/1(Out1) -> EPS_ConcussAvailabilityStatus_Convert/1
  EPS_ConcussAvailabilityStatus_Convert/1 -> EPS_ConcussAvailabilityStatus_L/1
  EPS_ConcussAvailabilityStatus_L/1 -> EPS_ConcussAvailabilityStatus_S/1
  EPS_ConcussAvailabilityStatus_S/1 -> EPS_ConcussAvailabilityStatuscv/1
  EPS_ConcussAvailabilityStatuscv/1 -> EPS_ConcussAvailabilityStatus_F/1
  EPS_Checksum_F/1 -> EPS_Checksum_Ad/1
  EPS_Checksum_O/1 -> EPS_Checksum_Ad/2
  EPS_Checksum_Ad/1 -> EPS_Checksum_sat/1
  EPS_Checksum_sat/1 -> EPS_Checksum_Out/1
  Demux/8 -> EPS_Checksum_Sub/1(In1)
  EPS_Checksum_Sub/1(Out1) -> EPS_Checksum_Convert/1
  EPS_Checksum_Convert/1 -> EPS_Checksum_L/1
  EPS_Checksum_L/1 -> EPS_Checksum_S/1
  EPS_Checksum_S/1 -> EPS_Checksumcv/1
  EPS_Checksumcv/1 -> EPS_Checksum_F/1
  input/1 -> Demux/1

== system VCU_CS75_12_16_Test/长安CS75底盘程序，20ms一次/Input/CAN1_Rx/EPS_21A/ReceiveMessages/Subsystem/EPS_21A2 ==
  input : Inport
  CRC_Ad : Sum
  CRC_Convert : DataTypeConversion  OutDataTypeStr=uint32
  CRC_F : Gain
  CRC_L : simulink/Logic and Bit Operations/Bitwise Operator  logicop=AND  UseBitMask=on  BitMask=255  BitMaskRealWorld=Stored Integer
  CRC_O : Constant  Value=0  OutDataTypeStr=single
  CRC_S : ArithShift
  CRC_Sub : Subsystem
  CRC_sat : Saturate  UpperLimit=0  LowerLimit=0
  CRCcv : DataTypeConversion
  Demux : Demux  Outputs=8
  EPS_AvailabilityStatus_Ad : Sum
  EPS_AvailabilityStatus_Convert : DataTypeConversion  OutDataTypeStr=uint32
  EPS_AvailabilityStatus_F : Gain
  EPS_AvailabilityStatus_L : simulink/Logic and Bit Operations/Bitwise Operator  logicop=AND  UseBitMask=on  BitMask=28  BitMaskRealWorld=Stored Integer
  EPS_AvailabilityStatus_O : Constant  Value=0  OutDataTypeStr=single
  EPS_AvailabilityStatus_S : ArithShift  BitShiftNumber=2
  EPS_AvailabilityStatus_Sub : Subsystem
  EPS_AvailabilityStatus_sat : Saturate  UpperLimit=7  LowerLimit=0
  EPS_AvailabilityStatuscv : DataTypeConversion
  EPS_IACC_abortReson_Ad : Sum
  EPS_IACC_abortReson_Convert : DataTypeConversion  OutDataTypeStr=uint32
  EPS_IACC_abortReson_F : Gain
  EPS_IACC_abortReson_L : simulink/Logic and Bit Operations/Bitwise Operator  logicop=AND  UseBitMask=on  BitMask=112  BitMaskRealWorld=Stored Integer
  EPS_IACC_abortReson_O : Constant  Value=0  OutDataTypeStr=single
  EPS_IACC_abortReson_S : ArithShift  BitShiftNumber=4
  EPS_IACC_abortReson_Sub : Subsystem
  EPS_IACC_abortReson_sat : Saturate  UpperLimit=7  LowerLimit=0
  EPS_IACC_abortResoncv : DataTypeConversion
  EPS_MeasTsionBatTorquevalid_Ad : Sum
  EPS_MeasTsionBatTorquevalid_Convert : DataTypeConversion  OutDataTypeStr=uint32
  EPS_MeasTsionBatTorquevalid_F : Gain
  EPS_MeasTsionBatTorquevalid_L : simulink/Logic and Bit Operations/Bitwise Operator  logicop=AND  UseBitMask=on  BitMask=64  BitMaskRealWorld=Stored Integer
  EPS_MeasTsionBatTorquevalid_O : Constant  Value=0  OutDataTypeStr=single
  EPS_MeasTsionBatTorquevalid_S : ArithShift  BitShiftNumber=6
  EPS_MeasTsionBatTorquevalid_Sub : Subsystem
  EPS_MeasTsionBatTorquevalid_sat : Saturate  UpperLimit=1  LowerLimit=0
  EPS_MeasTsionBatTorquevalidcv : DataTypeConversion
  EPS_MeasuredTosionBatTorque_Ad : Sum
  EPS_MeasuredTosionBatTorque_Convert : DataTypeConversion  OutDataTypeStr=uint32
  EPS_MeasuredTosionBatTorque_F : Gain  Gain=0.01
  EPS_MeasuredTosionBatTorque_L : simulink/Logic and Bit Operations/Bitwise Operator  logicop=AND  UseBitMask=on  BitMask=65504  BitMaskRealWorld=Stored Integer
  EPS_MeasuredTosionBatTorque_O : Constant  Value=-10.23  OutDataTypeStr=single
  EPS_MeasuredTosionBatTorque_S : ArithShift  BitShiftNumber=5
  EPS_MeasuredTosionBatTorque_Sub : Subsystem
  EPS_MeasuredTosionBatTorque_sat : Saturate  UpperLimit=10.23  LowerLimit=-10.23
  EPS_MeasuredTosionBatTorquecv : DataTypeConversion
  EPS_MeasuredTosionBatTorqueinput1_Ad : Sum
  EPS_MeasuredTosionBatTorqueinput1_C : Constant  Value=256
  EPS_MeasuredTosionBatTorqueinput1_P : Product
  Rollingcounter_Ad : Sum
  Rollingcounter_Convert : DataTypeConversion  OutDataTypeStr=uint32
  Rollingcounter_F : Gain
  Rollingcounter_L : simulink/Logic and Bit Operations/Bitwise Operator  logicop=AND  UseBitMask=on  BitMask=15  BitMaskRealWorld=Stored Integer
  Rollingcounter_O : Constant  Value=0  OutDataTypeStr=single
  Rollingcounter_S : ArithShift
  Rollingcounter_Sub : Subsystem
  Rollingcounter_sat : Saturate  UpperLimit=15  LowerLimit=0
  Rollingcountercv : DataTypeConversion
  EPS_MeasuredTosionBatTorque_Out : Outport
  EPS_AvailabilityStatus_Out : Outport  Port=2
  EPS_MeasTsionBatTorquevalid_Out : Outport  Port=3
  EPS_IACC_abortReson_Out : Outport  Port=4
  Rollingcounter_Out : Outport  Port=5
  CRC_Out : Outport  Port=6
  wires:
  EPS_MeasuredTosionBatTorque_F/1 -> EPS_MeasuredTosionBatTorque_Ad/1
  EPS_MeasuredTosionBatTorque_O/1 -> EPS_MeasuredTosionBatTorque_Ad/2
  EPS_MeasuredTosionBatTorque_Ad/1 -> EPS_MeasuredTosionBatTorque_sat/1
  EPS_MeasuredTosionBatTorque_sat/1 -> EPS_MeasuredTosionBatTorque_Out/1
  Demux/1 -> EPS_MeasuredTosionBatTorqueinput1_P/1
  EPS_MeasuredTosionBatTorqueinput1_C/1 -> EPS_MeasuredTosionBatTorqueinput1_P/2
  EPS_MeasuredTosionBatTorqueinput1_P/1 -> EPS_MeasuredTosionBatTorqueinput1_Ad/1
  Demux/2 -> EPS_MeasuredTosionBatTorqueinput1_Ad/2
  EPS_MeasuredTosionBatTorqueinput1_Ad/1 -> EPS_MeasuredTosionBatTorque_Sub/1(In1)
  EPS_MeasuredTosionBatTorque_Sub/1(Out1) -> EPS_MeasuredTosionBatTorque_Convert/1
  EPS_MeasuredTosionBatTorque_Convert/1 -> EPS_MeasuredTosionBatTorque_L/1
  EPS_MeasuredTosionBatTorque_L/1 -> EPS_MeasuredTosionBatTorque_S/1
  EPS_MeasuredTosionBatTorque_S/1 -> EPS_MeasuredTosionBatTorquecv/1
  EPS_MeasuredTosionBatTorquecv/1 -> EPS_MeasuredTosionBatTorque_F/1
  EPS_AvailabilityStatus_F/1 -> EPS_AvailabilityStatus_Ad/1
  EPS_AvailabilityStatus_O/1 -> EPS_AvailabilityStatus_Ad/2
  EPS_AvailabilityStatus_Ad/1 -> EPS_AvailabilityStatus_sat/1
  EPS_AvailabilityStatus_sat/1 -> EPS_AvailabilityStatus_Out/1
  Demux/3 -> EPS_AvailabilityStatus_Sub/1(In1)
  EPS_AvailabilityStatus_Sub/1(Out1) -> EPS_AvailabilityStatus_Convert/1
  EPS_AvailabilityStatus_Convert/1 -> EPS_AvailabilityStatus_L/1
  EPS_AvailabilityStatus_L/1 -> EPS_AvailabilityStatus_S/1
  EPS_AvailabilityStatus_S/1 -> EPS_AvailabilityStatuscv/1
  EPS_AvailabilityStatuscv/1 -> EPS_AvailabilityStatus_F/1
  EPS_MeasTsionBatTorquevalid_F/1 -> EPS_MeasTsionBatTorquevalid_Ad/1
  EPS_MeasTsionBatTorquevalid_O/1 -> EPS_MeasTsionBatTorquevalid_Ad/2
  EPS_MeasTsionBatTorquevalid_Ad/1 -> EPS_MeasTsionBatTorquevalid_sat/1
  EPS_MeasTsionBatTorquevalid_sat/1 -> EPS_MeasTsionBatTorquevalid_Out/1
  Demux/5 -> EPS_MeasTsionBatTorquevalid_Sub/1(In1)
  EPS_MeasTsionBatTorquevalid_Sub/1(Out1) -> EPS_MeasTsionBatTorquevalid_Convert/1
  EPS_MeasTsionBatTorquevalid_Convert/1 -> EPS_MeasTsionBatTorquevalid_L/1
  EPS_MeasTsionBatTorquevalid_L/1 -> EPS_MeasTsionBatTorquevalid_S/1
  EPS_MeasTsionBatTorquevalid_S/1 -> EPS_MeasTsionBatTorquevalidcv/1
  EPS_MeasTsionBatTorquevalidcv/1 -> EPS_MeasTsionBatTorquevalid_F/1
  EPS_IACC_abortReson_F/1 -> EPS_IACC_abortReson_Ad/1
  EPS_IACC_abortReson_O/1 -> EPS_IACC_abortReson_Ad/2
  EPS_IACC_abortReson_Ad/1 -> EPS_IACC_abortReson_sat/1
  EPS_IACC_abortReson_sat/1 -> EPS_IACC_abortReson_Out/1
  Demux/6 -> EPS_IACC_abortReson_Sub/1(In1)
  EPS_IACC_abortReson_Sub/1(Out1) -> EPS_IACC_abortReson_Convert/1
  EPS_IACC_abortReson_Convert/1 -> EPS_IACC_abortReson_L/1
  EPS_IACC_abortReson_L/1 -> EPS_IACC_abortReson_S/1
  EPS_IACC_abortReson_S/1 -> EPS_IACC_abortResoncv/1
  EPS_IACC_abortResoncv/1 -> EPS_IACC_abortReson_F/1
  Rollingcounter_F/1 -> Rollingcounter_Ad/1
  Rollingcounter_O/1 -> Rollingcounter_Ad/2
  Rollingcounter_Ad/1 -> Rollingcounter_sat/1
  Rollingcounter_sat/1 -> Rollingcounter_Out/1
  Demux/7 -> Rollingcounter_Sub/1(In1)
  Rollingcounter_Sub/1(Out1) -> Rollingcounter_Convert/1
  Rollingcounter_Convert/1 -> Rollingcounter_L/1
  Rollingcounter_L/1 -> Rollingcounter_S/1
  Rollingcounter_S/1 -> Rollingcountercv/1
  Rollingcountercv/1 -> Rollingcounter_F/1
  CRC_F/1 -> CRC_Ad/1
  CRC_O/1 -> CRC_Ad/2
  CRC_Ad/1 -> CRC_sat/1
  CRC_sat/1 -> CRC_Out/1
  Demux/8 -> CRC_Sub/1(In1)
  CRC_Sub/1(Out1) -> CRC_Convert/1
  CRC_Convert/1 -> CRC_L/1
  CRC_L/1 -> CRC_S/1
  CRC_S/1 -> CRCcv/1
  CRCcv/1 -> CRC_F/1
  input/1 -> Demux/1
